simulink subsystem "PvtSubSys_VSM_TSR"  (R2020b)
settings: Solver=VariableStepAuto  StartTime=0.0  StopTime=10.0  RelTol=1e-3
values from neighbouring files (symbols this model uses):
  P_VSM_TSR_Dis_keep_SPL_Table : value not decoded    [TSR.sldd]
  P_VSM_TSR_Dis_keep_SPLend = 50.0    [TSR.sldd]
  P_VSM_TSR_Dis_keep_TS_Table : value not decoded    [TSR.sldd]
  P_VSM_TSR_Ena_SPLSupp_Table : value not decoded    [TSR.sldd]
  P_VSM_TSR_Ena_TS_Table : value not decoded    [TSR.sldd]
  P_VSM_TSR_SLIF_Speed_High = 150.0    [TSR.sldd]
  P_VSM_TSR_SLIF_Speed_Low = 0.0    [TSR.sldd]
  P_VSM_TSR_SLW_SnvtySwitch = 0.0    [TSR.sldd]
  P_VSM_TSR_SLW_Speed_Delta_disable = 1.0    [TSR.sldd]
  P_VSM_TSR_SLW_Speed_Delta_enable = 0.0    [TSR.sldd]
  P_VSM_TSR_SLW_Speed_High = 150.0    [TSR.sldd]
  P_VSM_TSR_SLW_Speed_Low = 30.0    [TSR.sldd]
  P_VSM_TSR_SLW_TrafEyeAvtiveDist = 100.0    [TSR.sldd]
  P_VSM_TSR_SLW_Warning_Time = 10.0    [TSR.sldd]
  P_VSM_TSR_SteerWheelAngle = 360.0    [TSR.sldd]
  P_VSM_TSR_SWS_speed_withDir = 9.0    [TSR.sldd]
  P_VSM_TSR_SWS_speed_woDir = 24.0    [TSR.sldd]
libraries: simulink x23
(part 2 of 2)

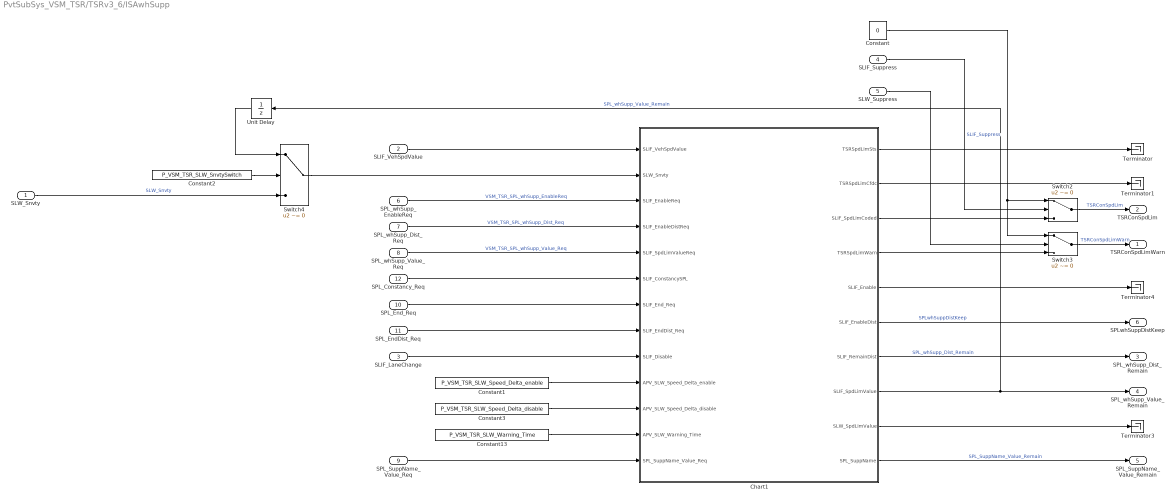
== system PvtSubSys_VSM_TSR/TSRv3_6/ISAwhSupp ==
  SLW_Snvty : Inport  OutDataTypeStr=single
  SLIF_VehSpdValue : Inport  Port=2
  SLIF_LaneChange : Inport  Port=3  OutDataTypeStr=boolean
  SLIF_Suppress : Inport  Port=4  OutDataTypeStr=boolean
  SLW_Suppress : Inport  Port=5
  SPL_whSupp_EnableReq : Inport  Port=6  OutDataTypeStr=boolean
  SPL_whSupp_Dist_Req : Inport  Port=7  OutDataTypeStr=single
  SPL_whSupp_Value_Req : Inport  Port=8  OutDataTypeStr=uint8
  SPL_SuppName_Value_Req : Inport  Port=9  OutDataTypeStr=uint8
  SPL_End_Req : Inport  Port=10  OutDataTypeStr=boolean
  SPL_EndDist_Req : Inport  Port=11  OutDataTypeStr=single
  SPL_Constancy_Req : Inport  Port=12  OutDataTypeStr=uint8
  Chart1 : Stateflow chart  TreatAsAtomicUnit=on
  Constant : Constant  Value=0  OutDataTypeStr=Inherit: Inherit via back propagation
  Constant1 : Constant  Value=P_VSM_TSR_SLW_Speed_Delta_enable
  Constant13 : Constant  Value=P_VSM_TSR_SLW_Warning_Time
  Constant2 : Constant  Value=P_VSM_TSR_SLW_SnvtySwitch
  Constant3 : Constant  Value=P_VSM_TSR_SLW_Speed_Delta_disable
  Switch2 : Switch  Criteria=u2 ~= 0
  Switch3 : Switch  Criteria=u2 ~= 0
  Switch4 : Switch  Criteria=u2 ~= 0  OutDataTypeStr=single
  Terminator{,1,3..4} (4 alike) : Terminator
  Unit Delay : UnitDelay  SampleTime=-1  HasFrameUpgradeWarning=on
  TSRConSpdLimWarn : Outport
  TSRConSpdLim : Outport  Port=2
  SPL_whSupp_Dist_Remain : Outport  Port=3  OutDataTypeStr=single
  SPL_whSupp_Value_Remain : Outport  Port=4  OutDataTypeStr=uint8
  SPL_SuppName_Value_Remain : Outport  Port=5  OutDataTypeStr=uint8
  SPLwhSuppDistKeep : Outport  Port=6  OutDataTypeStr=single
  wires:
  Constant/1 -> Switch2/1, Switch3/1
  Chart1/2(TSRSpdLimCfdc) -> Terminator1/1
  Chart1/1(TSRSpdLimSts) -> Terminator/1
  SLW_Suppress/1 -> Switch3/2
  Chart1/4(TSRSpdLimWarn) -> Switch3/3
  Switch2/1 -> TSRConSpdLim/1  "TSRConSpdLim"
  Chart1/3(SLIF_SpdLimCoded) -> Switch2/3
  SPL_EndDist_Req/1 -> Chart1/8(SLIF_EndDist_Req)
  Chart1/6(SLIF_EnableDist) -> SPLwhSuppDistKeep/1  "SPLwhSuppDistKeep"
  Switch3/1 -> TSRConSpdLimWarn/1  "TSRConSpdLimWarn"
  Chart1/5(SLIF_Enable) -> Terminator4/1
  SPL_End_Req/1 -> Chart1/7(SLIF_End_Req)
  SPL_Constancy_Req/1 -> Chart1/6(SLIF_ConstancySPL)
  SLIF_Suppress/1 -> Switch2/2  "SLIF_Suppress"
  SPL_whSupp_EnableReq/1 -> Chart1/3(SLIF_EnableReq)  "VSM_TSR_SPL_whSupp_EnableReq"
  Chart1/7(SLIF_RemainDist) -> SPL_whSupp_Dist_Remain/1  "SPL_whSupp_Dist_Remain"
  SPL_whSupp_Value_Req/1 -> Chart1/5(SLIF_SpdLimValueReq)  "VSM_TSR_SPL_whSupp_Value_Req"
  SLIF_VehSpdValue/1 -> Chart1/1(SLIF_VehSpdValue)
  SPL_whSupp_Dist_Req/1 -> Chart1/4(SLIF_EnableDistReq)  "VSM_TSR_SPL_whSupp_Dist_Req"
  Chart1/10(SPL_SuppName) -> SPL_SuppName_Value_Remain/1  "SPL_SuppName_Value_Remain"
  SLIF_LaneChange/1 -> Chart1/9(SLIF_Disable)
  Chart1/9(SLW_SpdLimValue) -> Terminator3/1
  SPL_SuppName_Value_Req/1 -> Chart1/13(SPL_SuppName_Value_Req)
  Constant1/1 -> Chart1/10(APV_SLW_Speed_Delta_enable)
  Constant3/1 -> Chart1/11(APV_SLW_Speed_Delta_disable)
  Constant13/1 -> Chart1/12(APV_SLW_Warning_Time)
  Constant2/1 -> Switch4/2
  Chart1/8(SLIF_SpdLimValue) -> Unit Delay/1, SPL_whSupp_Value_Remain/1  "SPL_whSupp_Value_Remain"
  Switch4/1 -> Chart1/2(SLW_Snvty)
  SLW_Snvty/1 -> Switch4/3  "SLW_Snvty"
  Unit Delay/1 -> Switch4/1

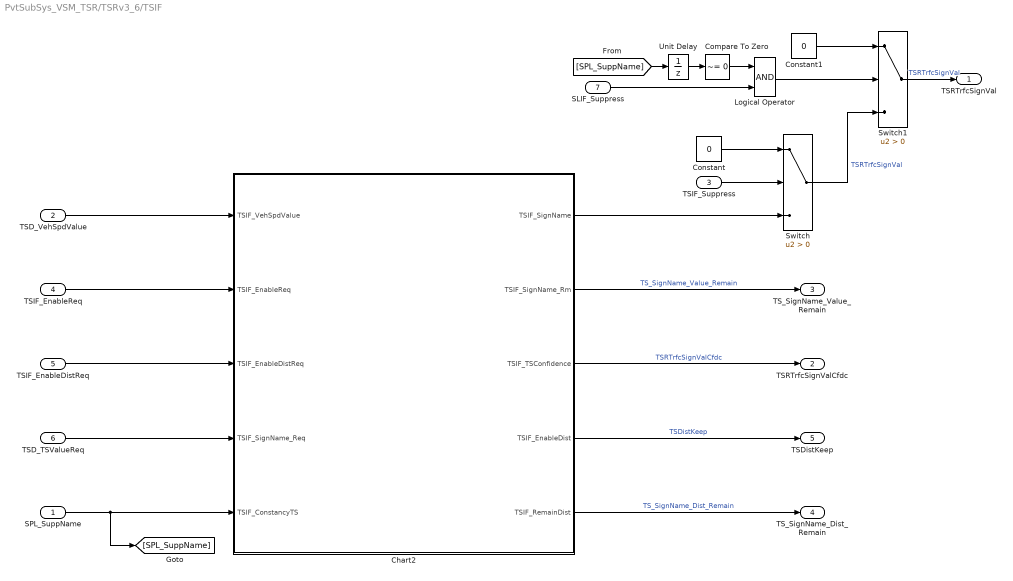
== system PvtSubSys_VSM_TSR/TSRv3_6/TSIF ==
  SPL_SuppName : Inport
  TSD_VehSpdValue : Inport  Port=2
  TSIF_Suppress : Inport  Port=3
  TSIF_EnableReq : Inport  Port=4  OutDataTypeStr=boolean
  TSIF_EnableDistReq : Inport  Port=5  OutDataTypeStr=single
  TSD_TSValueReq : Inport  Port=6  OutDataTypeStr=uint8
  SLIF_Suppress : Inport  Port=7
  Chart2 : Stateflow chart  TreatAsAtomicUnit=on
  Compare To Zero : simulink/Logic and Bit Operations/Compare To Zero  relop=~=  OutDataTypeStr=boolean
  Constant : Constant  Value=0  OutDataTypeStr=Inherit: Inherit via back propagation
  Constant1 : Constant  Value=0  OutDataTypeStr=Inherit: Inherit via back propagation
  Logical Operator : Logic  AllPortsSameDT=off  OutDataTypeStr=boolean
  Switch : Switch  Criteria=u2 > Threshold
  Switch1 : Switch  Criteria=u2 > Threshold
  Unit Delay : UnitDelay  SampleTime=-1  HasFrameUpgradeWarning=on
  TSRTrfcSignVal : Outport
  TSRTrfcSignValCfdc : Outport  Port=2
  TS_SignName_Value_Remain : Outport  Port=3
  TS_SignName_Dist_Remain : Outport  Port=4
  TSDistKeep : Outport  Port=5
  wires:
  TSIF_EnableDistReq/1 -> Chart2/3(TSIF_EnableDistReq)
  TSIF_EnableReq/1 -> Chart2/2(TSIF_EnableReq)
  TSD_TSValueReq/1 -> Chart2/4(TSIF_SignName_Req)
  TSD_VehSpdValue/1 -> Chart2/1(TSIF_VehSpdValue)
  TSIF_Suppress/1 -> Switch/2
  SPL_SuppName/1 -> [SPL_SuppName], Chart2/5(TSIF_ConstancyTS)
  Chart2/3(TSIF_TSConfidence) -> TSRTrfcSignValCfdc/1  "TSRTrfcSignValCfdc"
  Chart2/5(TSIF_RemainDist) -> TS_SignName_Dist_Remain/1  "TS_SignName_Dist_Remain"
  Chart2/4(TSIF_EnableDist) -> TSDistKeep/1  "TSDistKeep"
  Chart2/2(TSIF_SignName_Rm) -> TS_SignName_Value_Remain/1  "TS_SignName_Value_Remain"
  Chart2/1(TSIF_SignName) -> Switch/3
  Switch/1 -> Switch1/3  "TSRTrfcSignVal"
  Constant/1 -> Switch/1
  SLIF_Suppress/1 -> Logical Operator/2
  [SPL_SuppName] -> Unit Delay/1
  Compare To Zero/1 -> Logical Operator/1
  Unit Delay/1 -> Compare To Zero/1
  Logical Operator/1 -> Switch1/2
  Constant1/1 -> Switch1/1
  Switch1/1 -> TSRTrfcSignVal/1  "TSRTrfcSignVal"

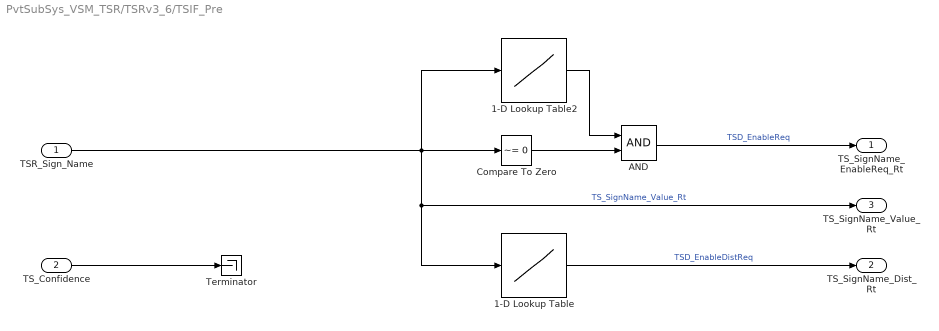
== system PvtSubSys_VSM_TSR/TSRv3_6/TSIF_Pre ==
  TSR_Sign_Name : Inport
  TS_Confidence : Inport  Port=2  OutDataTypeStr=single
  1-D Lookup Table : Lookup_n-D  NumberOfTableDimensions=1  BreakpointsForDimension1=[0:47]  BreakpointsForDimension1DataTypeStr=uint8  Table=P_VSM_TSR_Dis_keep_TS_Table  TableDataTypeStr=Inherit: Inherit from 'Table data'  InterpMethod=Nearest  InternalRulePriority=Speed  OutDataTypeStr=single  RndMeth=Simplest  InputSameDT=on
  1-D Lookup Table2 : Lookup_n-D  NumberOfTableDimensions=1  BreakpointsForDimension1=[0:47]  Table=P_VSM_TSR_Ena_TS_Table  TableDataTypeStr=Inherit: Inherit from 'Table data'  InterpMethod=Nearest  InternalRulePriority=Speed  RndMeth=Simplest  InputSameDT=on
  AND : Logic  AllPortsSameDT=off  OutDataTypeStr=boolean
  Compare To Zero : simulink/Logic and Bit Operations/Compare To Zero  relop=~=  OutDataTypeStr=boolean
  Terminator : Terminator
  TS_SignName_EnableReq_Rt : Outport
  TS_SignName_Dist_Rt : Outport  Port=2  OutDataTypeStr=single
  TS_SignName_Value_Rt : Outport  Port=3
  wires:
  TSR_Sign_Name/1 -> 1-D Lookup Table/1, TS_SignName_Value_Rt/1, 1-D Lookup Table2/1, Compare To Zero/1  "TS_SignName_Value_Rt"
  1-D Lookup Table/1 -> TS_SignName_Dist_Rt/1  "TSD_EnableDistReq"
  Compare To Zero/1 -> AND/2
  1-D Lookup Table2/1 -> AND/1
  AND/1 -> TS_SignName_EnableReq_Rt/1  "TSD_EnableReq"
  TS_Confidence/1 -> Terminator/1

== matlab function PvtSubSys_VSM_TSR/TSRv3_6/ISA_Pre/MATLAB Function ==
  data: SPL_noSupp_EnableReq input; SPL_noSupp_EnableReq_Rt output; SPL_noSupp_Value input; SPL_whSupp_EnableReq input; SPL_whSupp_Value input; SPL_noSupp_Value_Rt output
function [SPL_noSupp_EnableReq_Rt, SPL_noSupp_Value_Rt]= fcn(SPL_noSupp_EnableReq, SPL_noSupp_Value,SPL_whSupp_EnableReq,SPL_whSupp_Value)

if SPL_whSupp_EnableReq>0
    SPL_noSupp_EnableReq_Rt=SPL_whSupp_EnableReq;
    SPL_noSupp_Value_Rt=SPL_whSupp_Value;
else
    SPL_noSupp_EnableReq_Rt=SPL_noSupp_EnableReq;
    SPL_noSupp_Value_Rt=SPL_noSupp_Value;
end
end

== stateflow chart PvtSubSys_VSM_TSR/TSRv3_6/ISA_Set/Chart ==
  state Init
    Turn_Flag=0;
  state Active
    Turn_Flag=1;
    en:
    time=0;
    du:
    time=time+1
  state On
    en:
    Dis=0;
    du:
    Dis=Dis+Speed*0.02/3.6
  (default) -> Init
  Active -> Init [order 1] : [temp==0&&time>150]
  Init -> On : [temp>0]
  On -> Init [order 2] : [temp==0]
  On -> Active [order 1] : [Dis>20]
  Active -> On [order 2] : [temp>0&&time>150]
  data: Turn_Flag output uint8; Speed input single; temp input boolean; time local uint8; Dis local single

== stateflow chart PvtSubSys_VSM_TSR/TSRv3_6/ISAnoSupp/Chart1 ==
  state ConstancySPL
    SLIF_Enable=true;
    SLIF_SpdLimValue=SLIF_ConstancySPL;
    SLIF_SpdLimCoded=SLIF_SpdLimValue/5;
    SLIF_EnableDist=single(0);
    TSRSpdLimCfdc=uint8(2);
    SLW_SpdLimValue = uint8(single(SLIF_SpdLimValue) + SLW_Snvty);
    SLW_SpdEnterThresh= SLW_SpdLimValue + APV_SLW_Speed_Delta_enable;
    SLW_SpdExitThresh = SLW_SpdLimValue - APV_SLW_Speed_Delta_disable;
    du:
    SLW_Vehicle_Speed=SLIF_VehSpdValue*1.03+1.3-SLW_Snvty;
    state No_Warning
      du:TSRSpdLimWarn=false;
    state Warning
      en:i=0;
      du:i=i+1;
      TSRSpdLimWarn=true;
    state Enouth_Warning
      du:TSRSpdLimWarn=false;
    ConstancySPL.Warning -> ConstancySPL.No_Warning [order 1] : [SLW_Vehicle_Speed<=SLW_SpdExitThresh]
    (default) -> ConstancySPL.No_Warning
    ConstancySPL.No_Warning -> ConstancySPL.Warning : [SLW_Vehicle_Speed>SLW_SpdEnterThresh]
    ConstancySPL.Enouth_Warning -> ConstancySPL.No_Warning : [SLW_Vehicle_Speed<=SLW_SpdExitThresh]
    ConstancySPL.Warning -> ConstancySPL.Enouth_Warning [order 2] : [(i>(APV_SLW_Warning_Time/0.02))]
  state SPLend
    en:
    SLIF_SPLendTotalDist=single(0);
    SLIF_RemainDist=single(0);
    SLIF_EndDist=SLIF_EndDist_Req;
    TSRSpdLimWarn=false;
    SLIF_SpdLimValue=uint8(0);
    SLIF_SpdLimCoded=uint8(0);
    TSRSpdLimSts=uint8(2);
    SLW_SpdLimValue=uint8(0);
    du:
    SLIF_SPLendTotalDist=SLIF_SPLendTotalDist+SLIF_VehSpdValue*0.02/3.6;
    ex:
    SLIF_SPLendTotalDist=single(0);
  state Disable
    SLIF_Enable=false;
    SLIF_SpdLimValue=uint8(0);
    SLIF_EnableDist=single(0);
    TSRSpdLimSts=uint8(0);
    TSRSpdLimCfdc=uint8(0);
    SLIF_SpdLimCoded=uint8(0);
    SPL_SuppName=uint8(0);
    TSRSpdLimWarn=false;
    SLW_SpdLimValue=uint8(0);
  state SPL
    en:m=0;
    du:m=m+1;
    state Ready
      SLIF_SpdLimValue=SLIF_SpdLimValueReq;
      SLIF_EnableDist=SLIF_EnableDistReq;
      SLIF_SPLTotalDist=0;
      SPL_SuppName=SPL_SuppName_Value_Req;
    state Enable
      en:
      TSRSpdLimSts=uint8(1);
      TSRSpdLimCfdc=uint8(2);
      SLIF_SpdLimCoded=SLIF_SpdLimValue/5;
      SLIF_Enable=true;
      SLW_SpdLimValue =uint8(single (SLIF_SpdLimValue) + SLW_Snvty);
      SLW_SpdEnterThresh= SLW_SpdLimValue + APV_SLW_Speed_Delta_enable;
      SLW_SpdExitThresh = SLW_SpdLimValue - APV_SLW_Speed_Delta_disable;
      du:
      SLIF_SPLTotalDist=SLIF_SPLTotalDist+SLIF_VehSpdValue*0.02/3.6;
      SLIF_RemainDist=SLIF_EnableDist-SLIF_SPLTotalDist;
      SLW_Vehicle_Speed=SLIF_VehSpdValue*1.03+1.3;
      state No_Warning
        du:TSRSpdLimWarn=false;
      state Warning
        en:i=0;
        du:i=i+1;
        TSRSpdLimWarn=true;
      state Enouth_Warning
        du:TSRSpdLimWarn=false;
      SPL.Enable.Warning -> SPL.Enable.No_Warning [order 1] : [SLW_Vehicle_Speed<=SLW_SpdExitThresh]
      (default) -> SPL.Enable.No_Warning
      SPL.Enable.No_Warning -> SPL.Enable.Warning : [SLW_Vehicle_Speed>SLW_SpdEnterThresh]
      SPL.Enable.Enouth_Warning -> SPL.Enable.No_Warning : [SLW_Vehicle_Speed<=SLW_SpdExitThresh]
      SPL.Enable.Warning -> SPL.Enable.Enouth_Warning [order 2] : [(i>(uint16(APV_SLW_Warning_Time)/0.02))]
    (default) -> Ready
    Enable -> Ready : [SLIF_EnableReq]
    Ready -> Enable : [~SLIF_EnableReq]
  ConstancySPL -> Disable [order 1] : [(SLIF_ConstancySPL==0)...
      | &&(~SLIF_EnableReq)]
  Disable -> ConstancySPL [order 2] : [SLIF_ConstancySPL~=0]
  ConstancySPL -> SPLend [order 3] : [SLIF_End_Req]
  ConstancySPL -> SPL [order 2] : [SLIF_EnableReq]
  (default) -> Disable
  SPLend -> Disable [order 2] : [SLIF_SPLendTotalDist>SLIF_EnableDist]
  SPL -> Disable [order 1] : [SLIF_SPLTotalDist>=SLIF_EnableDist...
      | ||SLIF_Disable]
  Disable -> SPL [order 1] : [SLIF_EnableReq]
  SPL -> SPLend [order 2] : [SLIF_End_Req&&m>250]
  SPLend -> SPL [order 1] : [SLIF_EnableReq]
  data: TSRSpdLimSts output; TSRSpdLimCfdc output; SLIF_SpdLimCoded output uint8; TSRSpdLimWarn output; SLIF_Enable output boolean; SLIF_VehSpdValue input; SLW_Snvty input; SLIF_EnableReq input; SLIF_EnableDistReq input single; SLIF_EnableDist output single; SLIF_RemainDist output single; SLIF_SpdLimValue output uint8; SLIF_SpdLimValueReq input uint8; SLIF_ConstancySPL input uint8; i local; SLW_SpdEnterThresh local; SLW_SpdExitThresh local; SLW_Vehicle_Speed local; SLW_SpdLimValue output; SLIF_SPLTotalDist local single; SLIF_End_Req input boolean; SLIF_EndDist_Req input single; SLIF_SPLendTotalDist local single; SLIF_EndDist local single; SLIF_Disable input; APV_SLW_Speed_Delta_enable input; APV_SLW_Speed_Delta_disable input; APV_SLW_Warning_Time input; SLIF_SpdLimValue_Hold local uint8; SPL_SuppName_Value_Req input uint8; SPL_SuppName output uint8; m local

== stateflow chart PvtSubSys_VSM_TSR/TSRv3_6/ISAwhSupp/Chart1 ==
  state ConstancySPL
    SLIF_Enable=true;
    SLIF_SpdLimValue=SLIF_ConstancySPL;
    SLIF_SpdLimCoded=SLIF_SpdLimValue/5;
    SLIF_EnableDist=single(0);
    TSRSpdLimCfdc=uint8(2);
    SLW_SpdLimValue = SLIF_SpdLimValue + uint8(SLW_Snvty);
    SLW_SpdEnterThresh= SLW_SpdLimValue + APV_SLW_Speed_Delta_enable;
    SLW_SpdExitThresh = SLW_SpdLimValue - APV_SLW_Speed_Delta_disable;
    du:
    SLW_Vehicle_Speed=SLIF_VehSpdValue*1.03+1.3-SLW_Snvty;
    state No_Warning
      du:TSRSpdLimWarn=false;
    state Warning
      en:i=0;
      du:i=i+1;
      TSRSpdLimWarn=true;
    state Enouth_Warning
      du:TSRSpdLimWarn=false;
    ConstancySPL.Warning -> ConstancySPL.No_Warning [order 1] : [SLW_Vehicle_Speed<=SLW_SpdExitThresh]
    (default) -> ConstancySPL.No_Warning
    ConstancySPL.No_Warning -> ConstancySPL.Warning : [SLW_Vehicle_Speed>SLW_SpdEnterThresh]
    ConstancySPL.Enouth_Warning -> ConstancySPL.No_Warning : [SLW_Vehicle_Speed<=SLW_SpdExitThresh]
    ConstancySPL.Warning -> ConstancySPL.Enouth_Warning [order 2] : [(i>(APV_SLW_Warning_Time/0.02))]
  state SPLend
    en:
    SLIF_SPLendTotalDist=single(0);
    SLIF_RemainDist=single(0);
    SLIF_EndDist=SLIF_EndDist_Req;
    TSRSpdLimWarn=false;
    SLIF_SpdLimValue=uint8(0);
    SLIF_SpdLimCoded=uint8(0);
    TSRSpdLimSts=uint8(2);
    du:
    SLIF_SPLendTotalDist=SLIF_SPLendTotalDist+SLIF_VehSpdValue*0.02/3.6;
    ex:
    SLIF_SPLendTotalDist=single(0);
  state Disable
    SLIF_Enable=false;
    SLIF_SpdLimValue=uint8(0);
    SLIF_EnableDist=single(0);
    TSRSpdLimSts=uint8(0);
    TSRSpdLimCfdc=uint8(0);
    SLIF_SpdLimCoded=uint8(0);
    SPL_SuppName=uint8(0);
    TSRSpdLimWarn=false;
  state SPL
    state Ready
      SLIF_SpdLimValue=SLIF_SpdLimValueReq;
      SLIF_EnableDist=SLIF_EnableDistReq;
      SLIF_SPLTotalDist=0;
      SPL_SuppName=SPL_SuppName_Value_Req;
    state Enable
      en:
      TSRSpdLimSts=uint8(1);
      TSRSpdLimCfdc=uint8(2);
      SLIF_SpdLimCoded=SLIF_SpdLimValue/5;
      SLIF_Enable=true;
      SLW_SpdLimValue = SLIF_SpdLimValue + uint8(SLW_Snvty);
      SLW_SpdEnterThresh= SLW_SpdLimValue + APV_SLW_Speed_Delta_enable;
      SLW_SpdExitThresh = SLW_SpdLimValue - APV_SLW_Speed_Delta_disable;
      du:
      SLIF_SPLTotalDist=SLIF_SPLTotalDist+SLIF_VehSpdValue*0.02/3.6;
      SLIF_RemainDist=SLIF_EnableDist-SLIF_SPLTotalDist;
      SLW_Vehicle_Speed=SLIF_VehSpdValue*1.03+1.3;
      state No_Warning
        du:TSRSpdLimWarn=false;
      state Warning
        en:i=0;
        du:i=i+1;
        TSRSpdLimWarn=true;
      state Enouth_Warning
        du:TSRSpdLimWarn=false;
      SPL.Enable.Warning -> SPL.Enable.No_Warning [order 1] : [SLW_Vehicle_Speed<=SLW_SpdExitThresh]
      (default) -> SPL.Enable.No_Warning
      SPL.Enable.No_Warning -> SPL.Enable.Warning : [SLW_Vehicle_Speed>SLW_SpdEnterThresh]
      SPL.Enable.Enouth_Warning -> SPL.Enable.No_Warning : [SLW_Vehicle_Speed<=SLW_SpdExitThresh]
      SPL.Enable.Warning -> SPL.Enable.Enouth_Warning [order 2] : [(i>(uint16(APV_SLW_Warning_Time)/0.02))]
    (default) -> Ready
    Enable -> Ready : [SLIF_EnableReq]
    Ready -> Enable : [~SLIF_EnableReq]
  ConstancySPL -> Disable [order 1] : [(SLIF_ConstancySPL==0)...
      | &&(~SLIF_EnableReq)]
  Disable -> ConstancySPL [order 2] : [SLIF_ConstancySPL~=0]
  ConstancySPL -> SPLend [order 3] : [SLIF_End_Req]
  ConstancySPL -> SPL [order 2] : [SLIF_EnableReq]
  (default) -> Disable
  SPLend -> Disable [order 2] : [SLIF_SPLendTotalDist>SLIF_EnableDist]
  SPL -> Disable [order 1] : [SLIF_SPLTotalDist>=SLIF_EnableDist...
      | ||SLIF_Disable]
  Disable -> SPL [order 1] : [SLIF_EnableReq]
  SPL -> SPLend [order 2] : [SLIF_End_Req]
  SPLend -> SPL [order 1] : [SLIF_EnableReq]
  data: TSRSpdLimSts output; TSRSpdLimCfdc output; SLIF_SpdLimCoded output uint8; TSRSpdLimWarn output; SLIF_Enable output boolean; SLIF_VehSpdValue input; SLW_Snvty input; SLIF_EnableReq input; SLIF_EnableDistReq input single; SLIF_EnableDist output single; SLIF_RemainDist output single; SLIF_SpdLimValue output uint8; SLIF_SpdLimValueReq input uint8; SLIF_ConstancySPL input uint8; i local; SLW_SpdEnterThresh local; SLW_SpdExitThresh local; SLW_Vehicle_Speed local; SLW_SpdLimValue output; SLIF_SPLTotalDist local single; SLIF_End_Req input boolean; SLIF_EndDist_Req input single; SLIF_SPLendTotalDist local single; SLIF_EndDist local single; SLIF_Disable input; APV_SLW_Speed_Delta_enable input; APV_SLW_Speed_Delta_disable input; APV_SLW_Warning_Time input; SLIF_SpdLimValue_Hold local uint8; SPL_SuppName_Value_Req input uint8; SPL_SuppName output uint8

== stateflow chart PvtSubSys_VSM_TSR/TSRv3_6/TSIF/Chart2 ==
  state ConstancyTS
    TSIF_SignName=TSIF_ConstancyTS+0x2f;
    TSIF_SignName_Rm=uint8(0);
    TSIF_EnableDist=single(0);
    TSIF_TSConfidence=uint8(2);
    TSIF_RemainDist=single(0);
  state Disable
    TSIF_SignName=uint8(0);
    TSIF_SignName_Rm=uint8(0);
    TSIF_EnableDist=single(0);
    TSIF_TSConfidence=uint8(0);
  state SPL
    state Ready
      TSIF_SignName=TSIF_SignName_Req;
      TSIF_SignName_Rm=TSIF_SignName_Req;
      TSIF_EnableDist=TSIF_EnableDistReq;
      TSIF_TSTotalDist=0;
    state Enable
      du:
      TSIF_TSTotalDist=TSIF_TSTotalDist+TSIF_VehSpdValue*0.02/3.6;
      TSIF_RemainDist=TSIF_EnableDist-TSIF_TSTotalDist;
      TSIF_TSConfidence=uint8(2);
    (default) -> Ready
    Enable -> Ready : [TSIF_EnableReq]
    Ready -> Enable : [~TSIF_EnableReq]
  ConstancyTS -> Disable : [TSIF_ConstancyTS==0]
  Disable -> ConstancyTS [order 2] : [TSIF_ConstancyTS~=0&&TSIF_EnableReq==0]
  SPL -> ConstancyTS [order 2] : [TSIF_ConstancyTS~=0]
  (default) -> Disable
  SPL -> Disable [order 1] : [TSIF_TSTotalDist>=TSIF_EnableDist]
  Disable -> SPL [order 1] : [TSIF_EnableReq]
  data: TSIF_SignName output uint8 size=1; TSIF_SignName_Rm output uint8 size=1; TSIF_TSConfidence output uint8 size=1; TSIF_VehSpdValue input single size=1; TSIF_EnableReq input boolean size=1; TSIF_EnableDistReq input single size=1; TSIF_EnableDist output single size=1; TSIF_RemainDist output single size=1; TSIF_SignName_Req input uint8 size=1; TSIF_ConstancyTS input uint8 size=1; TSIF_TSTotalDist local single size=1

== stateflow chart PvtSubSys_VSM_TSR/TSRv3_6/TSRSM ==
  state Start
  state INIT
    SPL_noSupp_Value_Req=SPL_noSupp_Value_Init;
    SPL_noSupp_Dist_Req=SPL_noSupp_Dist_Init;
    SPL_whSupp_Dist_Req=SPL_whSupp_Dist_Init;
    SPL_whSupp_Value_Req=SPL_whSupp_Value_Init;
    SPL_SuppName_Value_Req=SPL_SuppName_Value_Init;
    TS_Dist_Req=TS_Dist_Init;
    TS_SignName_Value_Req=TS_SignName_Value_Init;
    SPL_End_Req=false;
    SPL_EndDist_Req=single(0);
    SPL_Constancy_Req=uint8(0);
  state OFF
    TSRSts=uint8(0);
    SPL_noSupp_EnableReq=false;
    SPL_noSupp_Dist_Req=single(0);
    SPL_noSupp_Value_Req=uint8(0);
    SPL_whSupp_EnableReq=false;
    SPL_whSupp_Dist_Req=single(0);
    SPL_whSupp_Value_Req=uint8(0);
    SPL_SuppName_Value_Req=uint8(0);
    TS_EnableReq=false;
    TS_Dist_Req=single(0);
    TS_SignName_Value_Req=uint8(0);
    SPL_End_Req=false;
    SPL_EndDist_Req=single(0);
    SPL_Constancy_Req=uint8(0);
  state ERROR
    TSRSts=uint8(4);
    SPL_noSupp_EnableReq=false;
    SPL_noSupp_Dist_Req=single(0);
    SPL_noSupp_Value_Req=uint8(0);
    SPL_whSupp_EnableReq=false;
    SPL_whSupp_Dist_Req=single(0);
    SPL_whSupp_Value_Req=uint8(0);
    SPL_SuppName_Value_Req=uint8(0);
    TS_EnableReq=false;
    TS_Dist_Req=single(0);
    TS_SignName_Value_Req=uint8(0);
    SPL_End_Req=false;
    SPL_EndDist_Req=single(0);
    SPL_Constancy_Req=uint8(0);
  state ON
    TSRSts=FUSSts;
    SPL_noSupp_EnableReq=SPL_noSupp_EnableReq_Rt;
    SPL_noSupp_Dist_Req=SPL_noSupp_Dist_Rt;
    SPL_noSupp_Value_Req=SPL_noSupp_Value_Rt;
    SPL_whSupp_EnableReq=SPL_whSupp_EnableReq_Rt;
    SPL_whSupp_Dist_Req=SPL_whSupp_Dist_Rt;
    SPL_whSupp_Value_Req=SPL_whSupp_Value_Rt;
    SPL_SuppName_Value_Req=SPL_SuppName_Value_Rt;
    TS_EnableReq=TS_EnableReq_Rt;
    TS_Dist_Req=TS_Dist_Rt;
    TS_SignName_Value_Req=TS_SignName_Value_Rt;
    SPL_End_Req=SPL_End_Rt;
    SPL_EndDist_Req=SPL_EndDist_Rt;
    SPL_Constancy_Req=SPL_Constancy_Rt;
  (default) -> Start
  Start -> (junction 170) : [VehConfigTSR==1&&TSR_error~=3]
  (junction 170) -> (junction 171) [order 1] : [SPL_noSupp_Value_Init~=0]
  (junction 170) -> (junction 172) [order 2] : {SPL_noSupp_EnableReq=false;}
  (junction 171) -> (junction 172) : {SPL_noSupp_EnableReq=true;}
  (junction 172) -> (junction 180)
  (junction 180) -> (junction 179) [order 1] : [SPL_whSupp_Value_Init~=0]
  (junction 180) -> (junction 175) [order 2] : {SPL_whSupp_EnableReq=false;}
  (junction 179) -> (junction 175) : {SPL_whSupp_EnableReq=true;}
  (junction 175) -> (junction 212)
  (junction 212) -> (junction 213) [order 1] : [TS_SignName_Value_Init~=0]
  (junction 212) -> (junction 214) [order 2] : {TS_EnableReq=false;}
  (junction 213) -> (junction 214) : {TS_EnableReq=true;}
  (junction 214) -> INIT
  INIT -> OFF [order 3] : [TSR_error==3]
  INIT -> ERROR [order 2] : [TSR_error==1]
  INIT -> ON [order 1] : [TSR_error~=1&&TSR_error~=3]
  ERROR -> OFF [order 2] : [TSR_error==3]
  OFF -> ERROR [order 2] : [TSR_error==1]
  ERROR -> ON [order 1] : [TSR_error~=1&&...
      | TSR_error~=3]
  ON -> ERROR [order 2] : [TSR_error==1]
  OFF -> ON [order 1] : [TSR_error~=3&&TSR_error~=1]
  ON -> OFF [order 1] : [TSR_error==3]
  data: VehConfigTSR input uint8; TSR_error input uint8; FUSSts input uint8; TSRSts output uint8; SPL_noSupp_Value_Req output uint8; SPL_noSupp_Value_Init input uint8; SPL_noSupp_Dist_Init input single; SPL_whSupp_Value_Init input uint8; SPL_SuppName_Value_Init input uint8; SPL_whSupp_Dist_Init input single; TS_SignName_Value_Init input uint8; TS_Dist_Init input single; SPL_noSupp_EnableReq_Rt input boolean; SPL_noSupp_Dist_Req output single; SPL_whSupp_Value_Req output uint8; SPL_SuppName_Value_Req output uint8; SPL_whSupp_Dist_Req output single; TS_SignName_Value_Req output uint8; TS_Dist_Req output single; SPL_noSupp_Dist_Rt input single; SPL_noSupp_Value_Rt input uint8; SPL_whSupp_EnableReq_Rt input boolean; SPL_whSupp_Dist_Rt input single; SPL_whSupp_Value_Rt input uint8; SPL_SuppName_Value_Rt input uint8; SPL_End_Rt input boolean; SPL_EndDist_Rt input single; SPL_Constancy_Rt input uint8; TS_EnableReq_Rt input boolean; TS_Dist_Rt input single; TS_SignName_Value_Rt input uint8; SPL_noSupp_EnableReq output boolean; SPL_whSupp_EnableReq output boolean; TS_EnableReq output boolean; SPL_End_Req output boolean; SPL_EndDist_Req output single; SPL_Constancy_Req output uint8
